simulink model "PX4_angRate_controller_GAoptimization"  (R2023b)
settings: Solver=FixedStepAuto  StartTime=0.0  StopTime=StopTime  FixedStep=1/IMU_GYRO_RATE  RelTol=1e-3
undefined symbols (not defined in the file or in its folder): C, D, dgyro_cutoff, FF, flag_noise, gain_resolution, gyro_cutoff, I, i, IMU_GYRO_RATE, K, noise_amplitude, P, Q, R, step_value, windup_limit
libraries: cstblocks x2, dspfdesign x2
settings Model: PacingRate=447  Creator=JSheng  LastModifiedBy=sbazzocchi
settings SolverCC: AlgebraicLoopSolver=TrustRegion
settings DataIOCC: ReturnWorkspaceOutputs=off
settings DebuggingCC: AlgebraicLoopMsg=none  InheritedTsInSrcMsg=none  UnconnectedInputMsg=warning  UnconnectedOutputMsg=warning  UnconnectedLineMsg=warning  ArithmeticOperatorsInVariantConditions=warning
settings ModelReferenceCC: EnableRefExpFcnMdlSchedulingChecks=on
settings SFSimCC: CustomCodeUndefinedFunction=UseInterfaceOnly
settings RTWCC: DLArmComputeVersion=19.05

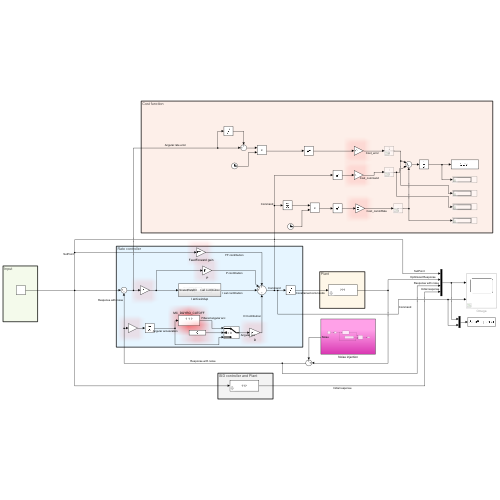
[thumbnail: Simulink's stored preview of the top-level diagram]
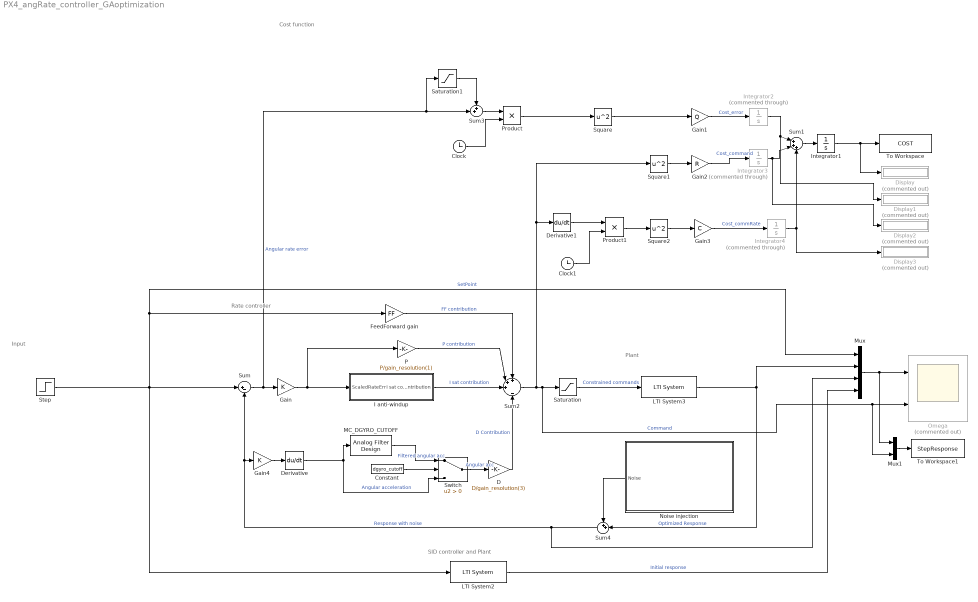
== system PX4_angRate_controller_GAoptimization ==
  note: Input
  note: SID controller and Plant
  note: Plant
  note: Cost function
  note: Rate controller
  Clock : Clock
  Clock1 : Clock
  Constant : Constant  Value=dgyro_cutoff
  D : Gain  Gain=D/gain_resolution(3)
  Derivative : Derivative  CoefficientInTFapproximation=1e10
  Derivative1 : Derivative
  Display{,1..3} (4 alike) : Display  Commented=on
  FeedForward gain : Gain  Gain=FF
  Gain : Gain  Gain=K
  Gain1 : Gain  Gain=Q
  Gain2 : Gain  Gain=R
  Gain3 : Gain  Gain=C
  Gain4 : Gain  Gain=K
  I anti-windup : Subsystem
  Integrator1 : Integrator
  Integrator2 : Integrator  Commented=through
  Integrator3 : Integrator  Commented=through
  Integrator4 : Integrator  Commented=through
  LTI System2 : cstblocks/LTI System  sys=G_temp  IC=[]  PadeOrder=0
  LTI System3 : cstblocks/LTI System  sys=A_temp  IC=[]  PadeOrder=0
  MC_DGYRO_CUTOFF : dspfdesign/Analog Filter Design  method=Butterworth  filttype=Lowpass  N=2  Wlo=max(1,dgyro_cutoff)*2*pi  Whi=80  Rp=2  Rs=40
  Mux : Mux
  Mux1 : Mux  Inputs=2
  Noise injection : Subsystem
      settings: PortSchema="{\"entries\":[{\"content\":{\"sides\":[{\"content\":{\"connectorIds\":[\"Out1\"]},\"type\":\"ConnectorPlacement.EquallySpacedRectSide\",\"uuid\":\"43dcf535-f749-446c-b8ed-9425fce616ea\"},{\"content\":{\"connectorIds\":[],\"side\":\"RIGHT\"},\"type\":\"ConnectorPlacement.EquallySpacedRectSide\",\"uuid\":\"b020978b-3129-44d5-aa5b-92d882fe7f2f\"},{\"content\":{\"connectorIds\":[],\"side\":\"TOP\"},\"type\":\"ConnectorPlacement.EquallySpacedRectSide\",\"uuid\":\"c027dc8d-5a89-443a-950b-22badb193d7a\"}]},\"type\":\"ConnectorPlacement.EquallySpacedConnector\",\"uuid\":\"402dbc5f-8df1-4001-8a00-9d04295efdf8\"}],\"packageUris\":[\"http://schema.mathworks.com/mf0/Connector/R2020b\"],\"version\":\"1.0\"}"
  "Omega " : Scope  Commented=on  NumInputPorts=2
  P : Gain  Gain=P/gain_resolution(1)
  Product : Product
  Product1 : Product
  Saturation : Saturate  UpperLimit=1  LowerLimit=-1
  Saturation1 : Saturate  UpperLimit=0  LowerLimit=-inf
  Square : Math  Operator=square
  Square1 : Math  Operator=square
  Square2 : Math  Operator=square
  Step : Step  After=step_value(i)
  Sum : Sum  Inputs=|+-
  Sum1 : Sum  Inputs=|+++
  Sum2 : Sum  Inputs=+++|-
  Sum3 : Sum  Inputs=++|
  Sum4 : Sum  Inputs=++|
  Switch : Switch  Criteria=u2 > Threshold  SaturateOnIntegerOverflow=off  InputSameDT=off
  To Workspace : ToWorkspace  VariableName=COST  SaveFormat=Timeseries  SampleTime=-1
  To Workspace1 : ToWorkspace  VariableName=StepResponse  SaveFormat=Timeseries  SampleTime=-1
  wires:
  Step/1 -> LTI System2/1, Mux/1, FeedForward gain/1, Sum/1  "SetPoint"
  Saturation/1 -> LTI System3/1  "Constrained commands"
  P/1 -> Sum2/2  "P contribution"
  Gain4/1 -> Derivative/1
  D/1 -> Sum2/4  "D Contribution"
  MC_DGYRO_CUTOFF/1 -> Switch/1  "Filtered angular acc"
  Sum/1 -> Saturation1/1, Sum3/2, Gain/1  "Angular rate error"
  LTI System2/1 -> Mux/4  "Initial response"
  FeedForward gain/1 -> Sum2/1  "FF contribution"
  Integrator1/1 -> Display/1, To Workspace/1
  Gain2/1 -> Integrator3/1  "Cost_command"
  Sum1/1 -> Integrator1/1
  Gain1/1 -> Integrator2/1  "Cost_error"
  Square1/1 -> Gain2/1
  Sum2/1 -> Mux1/2, "Omega "/2, Saturation/1, Square1/1, Derivative1/1  "Command"
  Derivative1/1 -> Product1/1
  Square2/1 -> Gain3/1
  Gain3/1 -> Integrator4/1  "Cost_commRate"
  Derivative/1 -> Switch/3, MC_DGYRO_CUTOFF/1  "Angular acceleration"
  LTI System3/1 -> Mux/2, Sum4/2  "Optimized Response"
  Integrator4/1 -> Sum1/3, Display3/1
  Integrator3/1 -> Sum1/2, Display2/1
  Integrator2/1 -> Display1/1, Sum1/1
  Square/1 -> Gain1/1
  Clock/1 -> Product/2
  Clock1/1 -> Product1/2
  Product1/1 -> Square2/1
  Product/1 -> Square/1
  Sum3/1 -> Product/1
  Saturation1/1 -> Sum3/1
  Sum4/1 -> Sum/2, Gain4/1, Mux/3  "Response with noise"
  Mux/1 -> Mux1/1, "Omega "/1
  Noise injection/1(Noise) -> Sum4/1
  Switch/1 -> D/1  "Angular acc"
  Constant/1 -> Switch/2
  Gain/1 -> P/1, I anti-windup/1(ScaledRateErr)
  I anti-windup/1(I sat contribution) -> Sum2/3  "I sat contribution"
  Mux1/1 -> To Workspace1/1

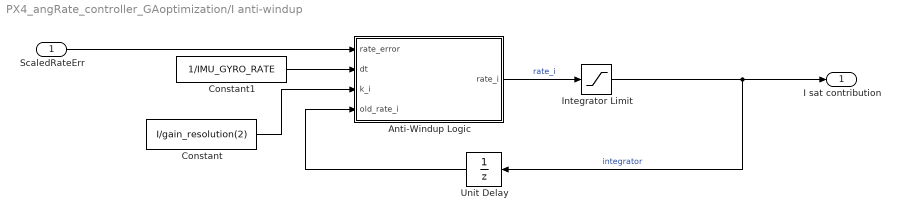
== system PX4_angRate_controller_GAoptimization/I anti-windup ==
  ScaledRateErr : Inport
  Anti-Windup Logic : MATLAB Function  TreatAsAtomicUnit=on
  Constant : Constant  Value=I/gain_resolution(2)
  Constant1 : Constant  Value=1/IMU_GYRO_RATE
  Integrator Limit : Saturate  UpperLimit=windup_limit  LowerLimit=-windup_limit
  Unit Delay : UnitDelay  SampleTime=-1  HasFrameUpgradeWarning=on
  I sat contribution : Outport
  wires:
  Integrator Limit/1 -> I sat contribution/1, Unit Delay/1  "integrator"
  Anti-Windup Logic/1(rate_i) -> Integrator Limit/1  "rate_i"
  Constant/1 -> Anti-Windup Logic/3(k_i)
  Constant1/1 -> Anti-Windup Logic/2(dt)
  ScaledRateErr/1 -> Anti-Windup Logic/1(rate_error)
  Unit Delay/1 -> Anti-Windup Logic/4(old_rate_i)

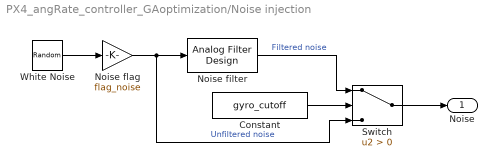
== system PX4_angRate_controller_GAoptimization/Noise injection ==
  Constant : Constant  Value=gyro_cutoff
  Noise filter : dspfdesign/Analog Filter Design  method=Butterworth  filttype=Lowpass  N=2  Wlo=max(1,gyro_cutoff)*2*pi  Whi=80  Rp=2  Rs=40
  Noise flag : Gain  Gain=flag_noise
  Switch : Switch  Criteria=u2 > Threshold  SaturateOnIntegerOverflow=off  InputSameDT=off
  White Noise : RandomNumber  Variance=noise_amplitude(i)
  Noise : Outport
  wires:
  Noise flag/1 -> Switch/3, Noise filter/1  "Unfiltered noise"
  White Noise/1 -> Noise flag/1
  Noise filter/1 -> Switch/1  "Filtered noise"
  Constant/1 -> Switch/2
  Switch/1 -> Noise/1

== matlab function PX4_angRate_controller_GAoptimization/I anti-windup/Anti-Windup Logic ==
  data: rate_error input; dt input; k_i input; rate_i output; old_rate_i input
function rate_i = fcn(rate_error, dt, k_i, old_rate_i)
    
   i_factor = rate_error/deg2rad(400);
   i_factor_sat = max(0, 1-i_factor*i_factor);
   rate_i=old_rate_i+i_factor_sat*k_i*rate_error*dt;
  

end
